simulink library "timecompensate"  (R2019b)
settings: Solver=VariableStepAuto  StartTime=0.0  StopTime=10.0  RelTol=1e-3

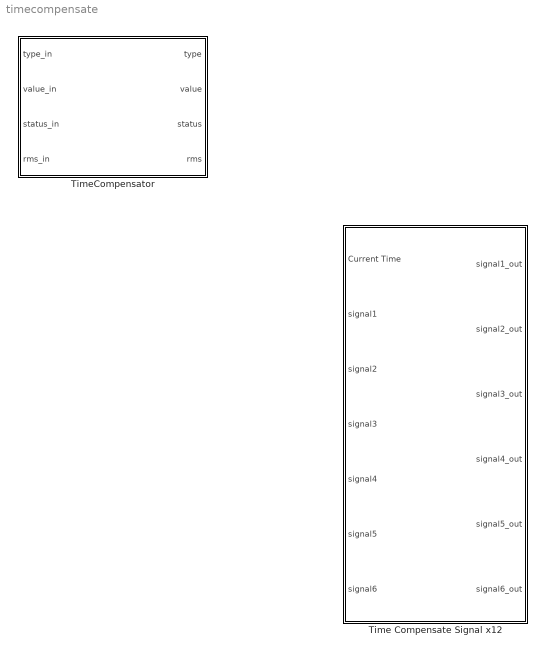
== system timecompensate ==
  Time Compensate Signal x12 : Subsystem
  TimeCompensator : MATLAB Function  TreatAsAtomicUnit=on

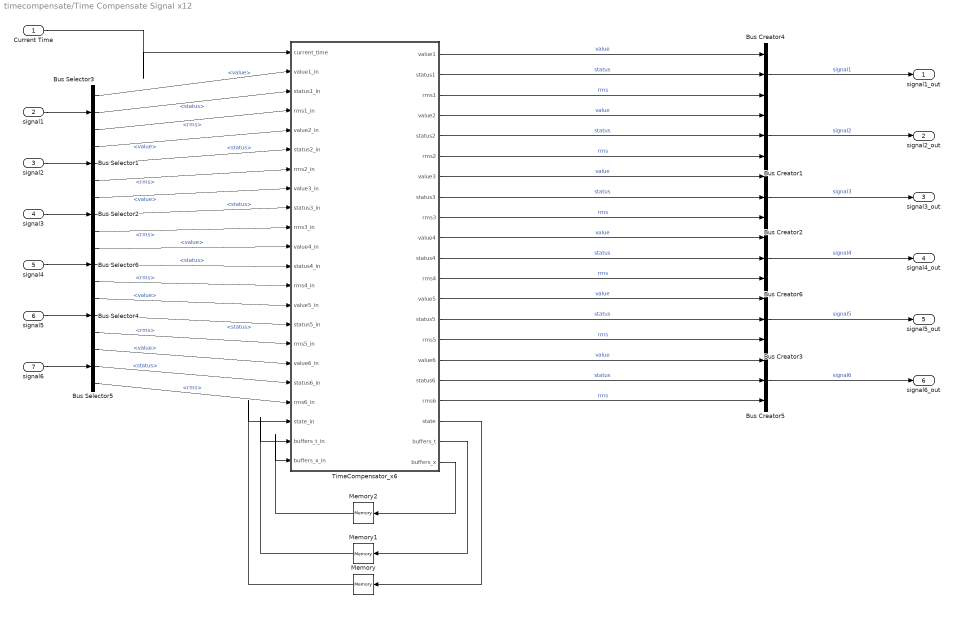
== system timecompensate/Time Compensate Signal x12 ==
  Current Time : Inport
  signal1 : Inport  Port=2  OutDataTypeStr=Bus: InputSignalObject
  signal2 : Inport  Port=3  OutDataTypeStr=Bus: InputSignalObject
  signal3 : Inport  Port=4  OutDataTypeStr=Bus: InputSignalObject
  signal4 : Inport  Port=5  OutDataTypeStr=Bus: InputSignalObject
  signal5 : Inport  Port=6  OutDataTypeStr=Bus: InputSignalObject
  signal6 : Inport  Port=7  OutDataTypeStr=Bus: InputSignalObject
  Bus Creator{1..6} (6 alike) : BusCreator  Inputs=3  OutDataTypeStr=Bus: OutputSignalObject  NonVirtualBus=on
  Bus Selector{1..6} (6 alike) : BusSelector  OutputSignals=value,status,rms
  Memory : Memory
  Memory1 : Memory
  Memory2 : Memory
  TimeCompensator_x6 : MATLAB Function  TreatAsAtomicUnit=on
  signal1_out : Outport
  signal2_out : Outport  Port=2
  signal3_out : Outport  Port=3
  signal4_out : Outport  Port=4
  signal5_out : Outport  Port=5
  signal6_out : Outport  Port=6
  wires:
  TimeCompensator_x6/14(status5) -> Bus Creator3/2  "status"
  TimeCompensator_x6/17(status6) -> Bus Creator5/2  "status"
  Bus Creator3/1 -> signal5_out/1  "signal5"
  Bus Creator6/1 -> signal4_out/1  "signal4"
  TimeCompensator_x6/18(rms6) -> Bus Creator5/3  "rms"
  TimeCompensator_x6/10(value4) -> Bus Creator6/1  "value"
  Bus Creator5/1 -> signal6_out/1  "signal6"
  TimeCompensator_x6/15(rms5) -> Bus Creator3/3  "rms"
  TimeCompensator_x6/13(value5) -> Bus Creator3/1  "value"
  TimeCompensator_x6/11(status4) -> Bus Creator6/2  "status"
  TimeCompensator_x6/16(value6) -> Bus Creator5/1  "value"
  TimeCompensator_x6/12(rms4) -> Bus Creator6/3  "rms"
  signal5/1 -> Bus Selector4/1
  signal4/1 -> Bus Selector6/1
  Bus Selector4/3 -> TimeCompensator_x6/16(rms5_in)  "<rms>"
  Bus Selector6/3 -> TimeCompensator_x6/13(rms4_in)  "<rms>"
  Bus Selector4/1 -> TimeCompensator_x6/14(value5_in)  "<value>"
  signal6/1 -> Bus Selector5/1
  Bus Selector4/2 -> TimeCompensator_x6/15(status5_in)  "<status>"
  Bus Selector5/3 -> TimeCompensator_x6/19(rms6_in)  "<rms>"
  Bus Selector5/1 -> TimeCompensator_x6/17(value6_in)  "<value>"
  Bus Selector6/2 -> TimeCompensator_x6/12(status4_in)  "<status>"
  Bus Selector5/2 -> TimeCompensator_x6/18(status6_in)  "<status>"
  Bus Selector6/1 -> TimeCompensator_x6/11(value4_in)  "<value>"
  TimeCompensator_x6/1(value1) -> Bus Creator4/1  "value"
  TimeCompensator_x6/8(status3) -> Bus Creator2/2  "status"
  Memory2/1 -> TimeCompensator_x6/22(buffers_x_in)
  TimeCompensator_x6/21(buffers_x) -> Memory2/1
  Bus Selector2/3 -> TimeCompensator_x6/10(rms3_in)  "<rms>"
  Bus Selector2/2 -> TimeCompensator_x6/9(status3_in)  "<status>"
  Bus Selector2/1 -> TimeCompensator_x6/8(value3_in)  "<value>"
  Memory1/1 -> TimeCompensator_x6/21(buffers_t_in)
  TimeCompensator_x6/20(buffers_t) -> Memory1/1
  Memory/1 -> TimeCompensator_x6/20(state_in)
  TimeCompensator_x6/19(state) -> Memory/1
  Bus Creator1/1 -> signal2_out/1  "signal2"
  Bus Creator4/1 -> signal1_out/1  "signal1"
  signal3/1 -> Bus Selector2/1
  signal2/1 -> Bus Selector1/1
  Bus Creator2/1 -> signal3_out/1  "signal3"
  signal1/1 -> Bus Selector3/1
  Current Time/1 -> TimeCompensator_x6/1(current_time)
  Bus Selector3/1 -> TimeCompensator_x6/2(value1_in)  "<value>"
  Bus Selector3/2 -> TimeCompensator_x6/3(status1_in)  "<status>"
  Bus Selector3/3 -> TimeCompensator_x6/4(rms1_in)  "<rms>"
  Bus Selector1/1 -> TimeCompensator_x6/5(value2_in)  "<value>"
  Bus Selector1/2 -> TimeCompensator_x6/6(status2_in)  "<status>"
  Bus Selector1/3 -> TimeCompensator_x6/7(rms2_in)  "<rms>"
  TimeCompensator_x6/2(status1) -> Bus Creator4/2  "status"
  TimeCompensator_x6/3(rms1) -> Bus Creator4/3  "rms"
  TimeCompensator_x6/4(value2) -> Bus Creator1/1  "value"
  TimeCompensator_x6/5(status2) -> Bus Creator1/2  "status"
  TimeCompensator_x6/6(rms2) -> Bus Creator1/3  "rms"
  TimeCompensator_x6/7(value3) -> Bus Creator2/1  "value"
  TimeCompensator_x6/9(rms3) -> Bus Creator2/3  "rms"

== matlab function timecompensate/Time Compensate Signal x12/TimeCompensator_x6 ==
function [value1,status1,rms1, ...
          value2,status2,rms2, ... 
          value3,status3,rms3, ...
          value4,status4,rms4, ...
          value5,status5,rms5, ...
          value6,status6,rms6, ...
          state,buffers_t,buffers_x]  = TimeCompensator_x6(current_time, ...
          value1_in,status1_in,rms1_in, ...
          value2_in,status2_in,rms2_in, ...
          value3_in,status3_in,rms3_in, ...
          value4_in,status4_in,rms4_in, ...
          value5_in,status5_in,rms5_in, ...
          value6_in,status6_in,rms6_in, ...
           state_in,buffers_t_in,buffers_x_in)
state = state_in;
buffers_t = buffers_t_in;
buffers_x = buffers_x_in;
if(state.initialized == 0)
    state.signal1_update_counter = uint32(1);
    state.signal2_update_counter = uint32(1);
    state.signal3_update_counter = uint32(1);
    state.signal4_update_counter = uint32(1);
    state.signal5_update_counter = uint32(1);
    state.signal6_update_counter = uint32(1);
    state.initialized = uint8(1);
else
     %buffers = buffers + 1;
end
index = 1;
[value1,status1,rms1,state.signal1_update_counter,buffers_x,buffers_t] = timecompensate_signal(...
    current_time,state.signal1_update_counter,index,value1_in,status1_in,rms1_in,buffers_x_in,buffers_t_in);
index = index + 1;
[value2,status2,rms2,state.signal2_update_counter,buffers_x,buffers_t] = timecompensate_signal(...
    current_time,state.signal2_update_counter,index,value2_in,status2_in,rms2_in,buffers_x_in,buffers_t_in);
index = index + 1;
[value3,status3,rms3,state.signal3_update_counter,buffers_x,buffers_t] = timecompensate_signal(...
    current_time,state.signal3_update_counter,index,value3_in,status3_in,rms3_in,buffers_x_in,buffers_t_in);
[value4,status4,rms4,state.signal4_update_counter,buffers_x,buffers_t] = timecompensate_signal(...
    current_time,state.signal4_update_counter,index,value4_in,status4_in,rms4_in,buffers_x_in,buffers_t_in);
index = index + 1;
[value5,status5,rms5,state.signal5_update_counter,buffers_x,buffers_t] = timecompensate_signal(...
    current_time,state.signal5_update_counter,index,value5_in,status5_in,rms5_in,buffers_x_in,buffers_t_in);
index = index + 1;
[value6,status6,rms6,state.signal6_update_counter,buffers_x,buffers_t] = timecompensate_signal(...
    current_time,state.signal6_update_counter,index,value6_in,status6_in,rms6_in,buffers_x_in,buffers_t_in);

== matlab function timecompensate/TimeCompensator ==
function [type,value,status,rms] = TimeCompensator(type_in,value_in,status_in,rms_in)

if(status_in == SignalState.SIGNALSTATE_UNDEFINED)
    value = 0;
    rms = 0;
    type = type_in;
    status = status_in;
elseif(status_in == SignalState.SIGNALSTATE_INITIALIZING)
    value = 0;
    rms = 0;
    type = type_in;
    status = status_in;
else
    value = value_in;
    rms = rms_in;
    type = type_in;
    status = status_in;
end
